simulink model "mracmsd"  (Simulink 7.0)
settings: Solver=ode45  StartTime=0.0  StopTime=10.0  RelTol=1e-3
values from neighbouring files (symbols this model uses):
  b = 2    [Mracini.m]
  bet0 = wn*wn    (= 100)    [Mracini.m]
  bet1 = 2*zeta*wn    (= 16)    [Mracini.m]
  gam1 = 100    [Mracini.m]
  gam2 = 10    [Mracini.m]
  m = 1    [Mracini.m]
libraries: simulink x1
settings Model: Creator=Kailu  LastModifiedBy=Kailu  ExtModeTrigMode=oneshot  ExtModeArmWhenConnect=off
settings DataIOCC: LimitDataPoints=off
settings OptimizationCC: BlockReduction=off  BooleanDataType=off
settings DebuggingCC: SaveWithParameterizedLinksMsg=none  SignalResolutionControl=TryResolveAllWithWarning  SolverPrmCheckMsg=none  MultiTaskDSMMsg=warning  MultiTaskCondExecSysMsg=none  StrictBusMsg=None
settings HardwareCC: TargetUnknown=on
settings RTWCC: IncludeERTFirstTime=on

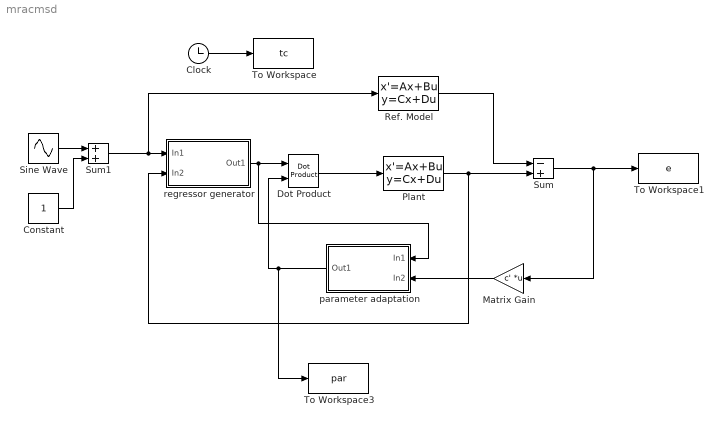
== system mracmsd ==
  Clock : Clock
      settings: Decimation=10
  Constant : Constant
  Dot Product : simulink/Math Operations/Dot Product  InputSameDT=on  OutDataType=sfix(16)  OutScaling=2^-10  DoSatur=off
  Matrix Gain : Gain  Orientation=left  Gain=c'  Multiplication=Matrix(K*u)  ParameterDataType=sfix(16)  ParameterScaling=2^0  OutDataType=sfix(16)  OutScaling=2^0  SaturateOnIntegerOverflow=on
  Plant : StateSpace  A=[0 1;0 -b/m]  B=[0;1/m]  C=[eye(2)]  D=zeros(2,1)
  Ref. Model : StateSpace  A=[0 1;-bet0 -bet1]  B=[0;bet0]  C=[eye(2)]  D=zeros(2,1)
  Sine Wave : Sin  Amplitude=0  Frequency=10  Phase=pi/2  SampleTime=0
  Sum : Sum  Inputs=-+  SaturateOnIntegerOverflow=on  InputSameDT=on
  Sum1 : Sum  SaturateOnIntegerOverflow=on  InputSameDT=on
  To Workspace : ToWorkspace  VariableName=tc  SampleTime=-1  SaveFormat=Array
  To Workspace1 : ToWorkspace  VariableName=e  SampleTime=-1  SaveFormat=Array
  To Workspace3 : ToWorkspace  VariableName=par  SampleTime=-1  SaveFormat=Array
  parameter adaptation : Subsystem  Orientation=left
  regressor generator : Subsystem
  wires:
  Matrix Gain/1 -> parameter adaptation/2(In2)
  Plant/1 -> regressor generator/2(In2), Sum/2
  Sum1/1 -> regressor generator/1(In1), Ref. Model/1
  Dot Product/1 -> Plant/1
  regressor generator/1(Out1) -> Dot Product/1, parameter adaptation/1(In1)
  Sine Wave/1 -> Sum1/1
  Constant/1 -> Sum1/2
  Clock/1 -> To Workspace/1
  parameter adaptation/1(Out1) -> Dot Product/2, To Workspace3/1
  Ref. Model/1 -> Sum/1
  Sum/1 -> Matrix Gain/1, To Workspace1/1

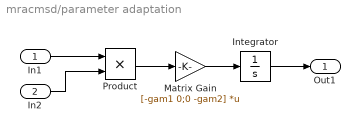
== system mracmsd/parameter adaptation ==
  In1 : Inport
  In2 : Inport  Port=2
  Integrator : Integrator
  Matrix Gain : Gain  Gain=[-gam1 0;0 -gam2]  Multiplication=Matrix(K*u)  ParameterDataType=sfix(16)  ParameterScaling=2^0  OutDataType=sfix(16)  OutScaling=2^0  SaturateOnIntegerOverflow=on
  Product : Product  SaturateOnIntegerOverflow=on  RndMeth=Zero  InputSameDT=on
  Out1 : Outport
  wires:
  In1/1 -> Product/1
  In2/1 -> Product/2
  Product/1 -> Matrix Gain/1
  Matrix Gain/1 -> Integrator/1
  Integrator/1 -> Out1/1

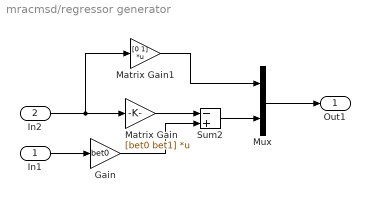
== system mracmsd/regressor generator ==
  In1 : Inport
  In2 : Inport  Port=2
  Gain : Gain  Gain=bet0  SaturateOnIntegerOverflow=on
  Matrix Gain : Gain  Gain=[bet0 bet1]  Multiplication=Matrix(K*u)  ParameterDataType=sfix(16)  ParameterScaling=2^0  OutDataType=sfix(16)  OutScaling=2^0  SaturateOnIntegerOverflow=on
  Matrix Gain1 : Gain  Gain=[0 1]  Multiplication=Matrix(K*u)  ParameterDataType=sfix(16)  ParameterScaling=2^0  OutDataType=sfix(16)  OutScaling=2^0  SaturateOnIntegerOverflow=on
  Mux : Mux  Inputs=2
  Sum2 : Sum  Inputs=-+  SaturateOnIntegerOverflow=on  InputSameDT=on
  Out1 : Outport
  wires:
  Mux/1 -> Out1/1
  Sum2/1 -> Mux/2
  Matrix Gain/1 -> Sum2/1
  In1/1 -> Gain/1
  Gain/1 -> Sum2/2
  In2/1 -> Matrix Gain/1, Matrix Gain1/1
  Matrix Gain1/1 -> Mux/1
